simulink model "Magnetometer"  (R2013a)
settings: Solver=ode3  SolverMode=SingleTasking  StartTime=0.0  StopTime=10.0  RelTol=1e-3
libraries: ZumoBotLib x2
settings Model: ExtModeTrigDuration=2  Creator=adesai  LastModifiedBy=cgupta
settings OptimizationCC: OptimizeModelRefInitCode=on  LifeSpan=1
settings DebuggingCC: SolverPrmCheckMsg=none  StrictBusMsg=Warning
settings HardwareCC: ProdBitPerInt=16  ProdBitPerPointer=8  ProdIntDivRoundTo=Zero  ProdEndianess=LittleEndian  ProdWordSize=8  ProdHWDeviceType=Atmel->AVR
settings RTWCC: SystemTargetFile=realtime.tlc  GenerateMakefile=off  TemplateMakefile=realtime.tmf  Description=Run on Target Hardware  RTWVerbose=off  ProcessScript=realtime_make_rtw_hook
settings STFCustomTargetCC: TargetLibSuffix=.a  GenerateSampleERTMain=on  ERTCustomFileBanners=on  SupportNonInlinedSFcns=off  SupportVariableSizeSignals=on  MATLABClassNameForMDSCustomization=Simulink.SoftwareTarget.ERTCustomization  SystemTargetFile=realtime.tlc
settings ERTTargetCC: ParMdlRefBuildCompliant=off  CompOptLevelCompliant=off  ConcurrentExecutionCompliant=off  CombineOutputUpdateFcns=off  ERTFirstTimeCompliant=off  SupportContinuousTime=on  SupportVariableSizeSignals=on  ModelStepFunctionPrototypeControlCompliant=off  CPPClassGenCompliant=off  ExtModeTransport=3  ExtModeMexFile=ext_serial_win32_comm  ExtModeMexArgs=0 1 9600  ERTSrcFileBannerTemplate=realtime_code_template.cgt  ERTHdrFileBannerTemplate=realtime_code_template.cgt  ERTDataSrcFileTemplate=realtime_code_template.cgt  ERTDataHdrFileTemplate=realtime_code_template.cgt  ERTCustomFileTemplate=realtime_file_process.tlc

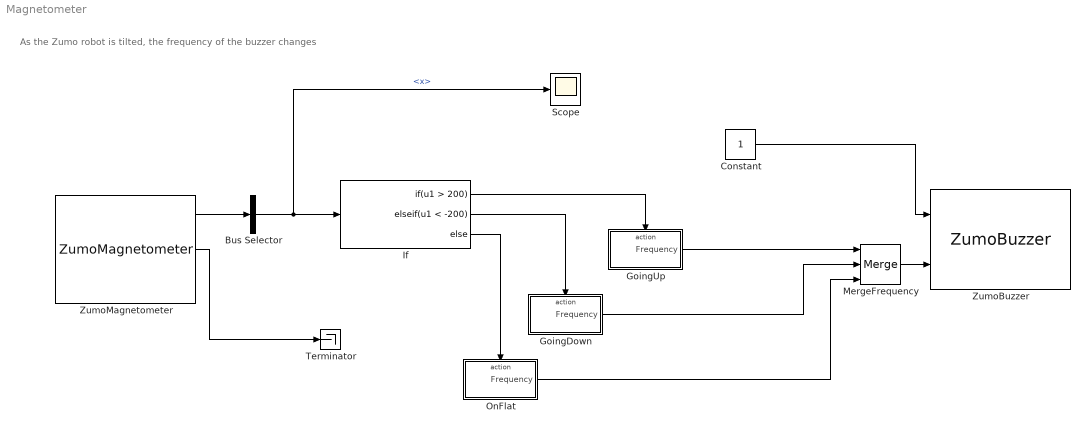
== system Magnetometer ==
  note: As the Zumo robot is tilted, the frequency
      | of the buzzer changes
  Bus Selector : BusSelector  OutputSignals=x
  Constant : Constant  OutDataTypeStr=boolean
  GoingDown : Subsystem  TreatAsAtomicUnit=on
  GoingUp : Subsystem  TreatAsAtomicUnit=on
  If : If  IfExpression=u1 > 200  ElseIfExpressions=u1 < -200
  MergeFrequency : Merge  Inputs=3
  OnFlat : Subsystem  TreatAsAtomicUnit=on
  Scope : Scope
  Terminator : Terminator
  ZumoBuzzer : ZumoBotLib/ZumoBuzzer
  ZumoMagnetometer : ZumoBotLib/ZumoMagnetometer  sampletime_lsm=0.02  debug_lsm=off  minX_lsm=-2048  maxX_lsm=2048  minY_lsm=-2048  maxY_lsm=2048  minZ_lsm=-4096  maxZ_lsm=4096
  wires:
  ZumoMagnetometer/1 -> Bus Selector/1
  Bus Selector/1 -> If/1, Scope/1  "<x>"
  ZumoMagnetometer/2 -> Terminator/1
  If/1 -> GoingUp/Action
  If/2 -> GoingDown/Action
  If/3 -> OnFlat/Action
  GoingUp/1(Frequency) -> MergeFrequency/1
  GoingDown/1(Frequency) -> MergeFrequency/2
  OnFlat/1(Frequency) -> MergeFrequency/3
  MergeFrequency/1 -> ZumoBuzzer/2
  Constant/1 -> ZumoBuzzer/1

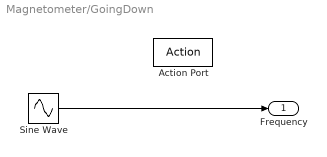
== system Magnetometer/GoingDown ==
  Action Port : ActionPort  ActionType=elseif
  Sine Wave : Sin  Amplitude=600  Bias=700
  Frequency : Outport
  wires:
  Sine Wave/1 -> Frequency/1

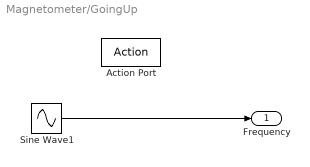
== system Magnetometer/GoingUp ==
  Action Port : ActionPort  ActionType=then
  Sine Wave1 : Sin  Amplitude=300  Bias=450
  Frequency : Outport
  wires:
  Sine Wave1/1 -> Frequency/1

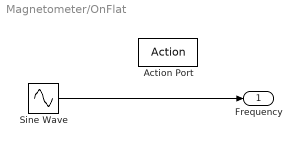
== system Magnetometer/OnFlat ==
  Action Port : ActionPort  ActionType=else
  Sine Wave : Sin  Amplitude=0
  Frequency : Outport
  wires:
  Sine Wave/1 -> Frequency/1
